simulink model "myDigPLL"  (Simulink 7.3)
settings: Solver=ode45  StartTime=0.0  StopTime=500*synM/synFr  FixedStep=1/(3*synFr*synN/synM)  MaxStep=.5/(synFr*synN/synM)  RelTol=1e-3
PreLoadFcn:
  | synM = 2230;    % frequency division ratio
  | synN = 1280*8;   % frequency division ratio
  | synFr = 217.77e6;   % reference frequency
  | synFq = 1e9;       % quiescent frequency
  | synSen = 40e6;   % VCO sensitivity
model workspace: external: M-Code (data not in the file)
libraries: commblksprivate x3, dsparch4 x1, commsynccomp2 x1
Description:
  | Phase-Locked Loop (PLL)  Based Frequency Synthesis
  | 
  | This demo shows how to simulate a phase-locked loop (PLL) frequency synthesizer.
CloseFcn:
  | clear synM synN synFr synFq synSen synSigsOut
settings Model: Creator=The MathWorks Inc.  LastModifiedBy=acarroll  CovMetricSettings=d  ExtModeAutoUpdateStatusClock=off
settings SolverCC: SignalSizeVariationType=Allow to vary during execution
settings DataIOCC: SaveOutput=off  SaveTime=off  SignalLoggingName=synSigsOut
settings OptimizationCC: BlockReduction=off  BooleanDataType=off  InlineInvariantSignals=on  InitFltsAndDblsToZero=on  EfficientMapNaN2IntZero=off
settings DebuggingCC: SaveWithParameterizedLinksMsg=none  CheckExecutionContextPreStartOutputMsg=on  CheckExecutionContextRuntimeOutputMsg=on  SignalResolutionControl=TryResolveAllWithWarning  SolverPrmCheckMsg=none  MultiTaskDSMMsg=warning  MultiTaskCondExecSysMsg=none  SigSpecEnsureSampleTimeMsg=none  StrictBusMsg=None
settings HardwareCC: TargetUnknown=on
settings ModelReferenceCC: UpdateModelReferenceTargets=IfOutOfDate
settings RTWCC: IncludeERTFirstTime=on
settings GRTTargetCC: TargetFcnLib=ansi_tfl_tmw.mat

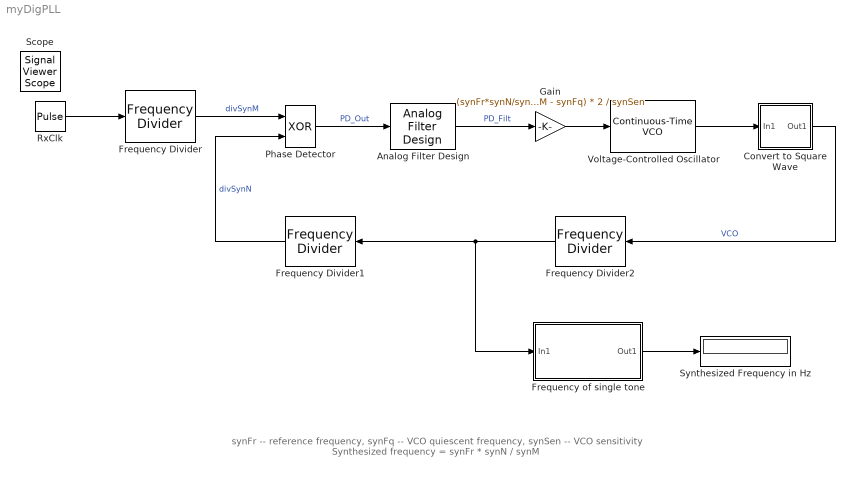
== system myDigPLL ==
  note: synFr -- reference frequency,  synFq -- VCO quiescent frequency,  synSen -- VCO sensitivity
      | Synthesized frequency = synFr * synN / synM
  Analog Filter Design : dsparch4/Analog Filter Design  method=Butterworth  filttype=Lowpass  N=1  Wlo=synFr/synM/10  Whi=80  Rp=2  Rs=40
  Convert to Square Wave : Subsystem
  Frequency Divider : commblksprivate/Frequency Divider  SystemSampleTime=-1  n=synM
  Frequency Divider1 : commblksprivate/Frequency Divider  SystemSampleTime=-1  n=1280
  Frequency Divider2 : commblksprivate/Frequency Divider  SystemSampleTime=-1  n=8
  Frequency of single tone : Subsystem
      mask Display: disp('Single Tone\nFrequency Estimator');
  Gain : Gain  Gain=(synFr*synN/synM - synFq) * 2 / synSen  ParameterDataType=sfix(16)  ParameterScaling=2^0  OutDataType=sfix(16)  OutScaling=2^0  SaturateOnIntegerOverflow=on  OutDataTypeStr=Inherit: Same as input  ParamDataTypeStr=Inherit: Same as input
  Phase Detector : Logic  Operator=XOR
  RxClk : DiscretePulseGenerator  PulseType=Time based  Amplitude=1  Period=1/synFr  PulseWidth=50  PhaseDelay=0  SampleTime=1
  Synthesized Frequency in Hz : Display
  Voltage-Controlled Oscillator : commsynccomp2/Continuous-Time VCO  SystemSampleTime=-1  Ac=1  Fc=synFq  Kc=synSen  Ph=0
  Scope : SignalViewerScope  IOType=viewer  NumInputPorts=4  ZoomMode=yonly  RefreshTime=0.018774
      settings: TimeRange=8.999999999999999e-005  YMin=-0.2~-0.2~-0.2~9.999999999999999e-005  YMax=1.2~1.2~1.2~0.0003  MaxDataPoints=500000
  wires:
  RxClk/1 -> Frequency Divider/1
  Phase Detector/1 -> Analog Filter Design/1  "PD_Out"
  Gain/1 -> Voltage-Controlled Oscillator/1
  Voltage-Controlled Oscillator/1 -> Convert to Square Wave/1(In1)
  Convert to Square Wave/1(Out1) -> Frequency Divider2/1  "VCO"
  Frequency Divider/1 -> Phase Detector/1  "divSynM"
  Frequency Divider1/1 -> Phase Detector/2  "divSynN"
  Analog Filter Design/1 -> Gain/1  "PD_Filt"
  Frequency of single tone/1(Out1) -> Synthesized Frequency in Hz/1
  Frequency Divider2/1 -> Frequency of single tone/1(In1), Frequency Divider1/1

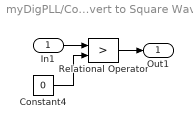
== system myDigPLL/Convert to Square Wave ==
  In1 : Inport  OutDataType=sfix(16)  OutScaling=2^0
  Constant4 : Constant  Value=0  OutDataType=sfix(16)  OutScaling=2^0
  Relational Operator : RelationalOperator  Operator=>  InputSameDT=on
  Out1 : Outport  OutDataType=sfix(16)  OutScaling=2^0
  wires:
  Relational Operator/1 -> Out1/1
  In1/1 -> Relational Operator/1
  Constant4/1 -> Relational Operator/2

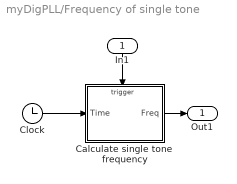
== system myDigPLL/Frequency of single tone ==
  In1 : Inport  OutDataType=sfix(16)  OutScaling=2^0
  Calculate single tone  frequency : Subsystem  TreatAsAtomicUnit=on
  Clock : Clock
  Out1 : Outport  OutDataType=sfix(16)  OutScaling=2^0
  wires:
  Calculate single tone  frequency/1(Freq) -> Out1/1
  Clock/1 -> Calculate single tone  frequency/1(Time)
  In1/1 -> Calculate single tone  frequency/Trigger

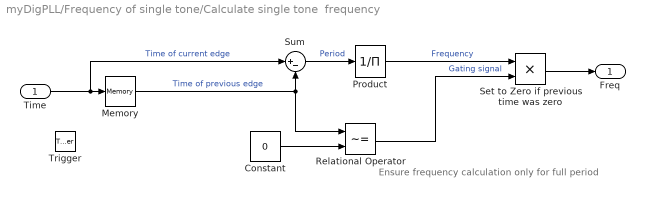
== system myDigPLL/Frequency of single tone/Calculate single tone  frequency ==
  note: Ensure frequency calculation
      | only for full period
  Time : Inport  OutDataType=sfix(16)  OutScaling=2^0
  Trigger : TriggerPort  ZeroCross=off
  Constant : Constant  Value=0  OutDataType=sfix(16)  OutScaling=2^0
  Memory : Memory  InheritSampleTime=on
  Product : Product  Inputs=/  OutDataType=sfix(16)  OutScaling=2^0  SaturateOnIntegerOverflow=on  InputSameDT=on  OutDataTypeStr=Inherit: Same as first input
  Relational Operator : RelationalOperator  Operator=~=  InputSameDT=on
  Set to Zero if previous time was zero : Product  OutDataType=sfix(16)  OutScaling=2^0  SaturateOnIntegerOverflow=on  InputSameDT=on  OutDataTypeStr=Inherit: Same as first input
  Sum : Sum  Inputs=|+-  OutDataType=sfix(16)  OutScaling=2^0  SaturateOnIntegerOverflow=on  InputSameDT=on  OutDataTypeStr=Inherit: Same as first input
  Freq : Outport  OutDataType=sfix(16)  OutScaling=2^0  InitialOutput=0
  wires:
  Relational Operator/1 -> Set to Zero if previous time was zero/2  "Gating signal"
  Constant/1 -> Relational Operator/2
  Set to Zero if previous time was zero/1 -> Freq/1
  Memory/1 -> Relational Operator/1, Sum/2  "Time of previous edge"
  Product/1 -> Set to Zero if previous time was zero/1  "Frequency"
  Sum/1 -> Product/1  "Period"
  Time/1 -> Memory/1, Sum/1  "Time of current edge"
